simulink model "MyMotorCU_RTW"  (Simulink 7.5)
settings: Solver=ode1  SolverMode=SingleTasking  StartTime=0.0  StopTime=inf  FixedStep=0.0002  RelTol=1e-3
PreLoadFcn:
  | vehicle = 'Car'; if ~length(which('cmcmd')), cmenv; end
  | MyMotorCU_RTW_bus
InitFcn:
  | vehicle = 'Car'; if ~length(which('cmcmd')), cmenv; end
  | MyMotorCU_RTW_bus
libraries: simulink x6
Description:
  | CarMaker Real-Time Target (generic)
settings Model: Creator=ml  LastModifiedBy=ml
settings DebuggingCC: SolverPrmCheckMsg=none
settings HardwareCC: TargetHWDeviceType=32-bit Generic  ProdEqTarget=off
settings RTWCC: SystemTargetFile=CarMaker.tlc  TemplateMakefile=CarMaker_unix.tmf  Description=CarMaker Real-Time Target (32-bit)  ProcessScript=CarMaker_make_rtw_hook
settings CodeAppCC: MaxIdLength=63
settings STFCustomTargetCC: ModelReferenceCompliant=off  GeneratePreprocessorConditionals=Disable all  SystemTargetFile=CarMaker.tlc
settings GRTTargetCC: ModelReferenceCompliant=off  ParMdlRefBuildCompliant=off  CompOptLevelCompliant=off  MatFileLogging=off  ExtModeMexFile=noextcomm
settings CustomProperty: DataType=string  Value=..
settings EnumStrPairs: String=Car

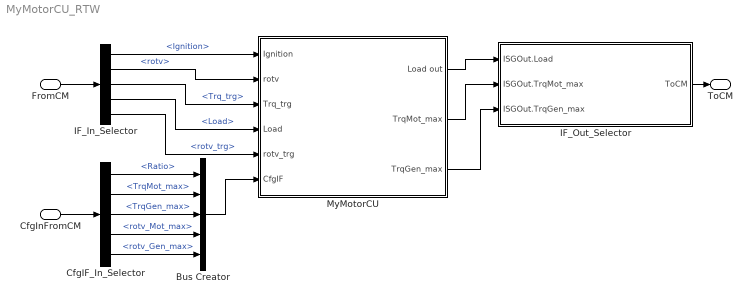
== system MyMotorCU_RTW ==
  FromCM : Inport  UseBusObject=on
      settings: BusObject=cmPTMotorCUIn
  CfgInFromCM : Inport  Port=2  UseBusObject=on
      settings: BusObject=cmPTMotorCUCfgIn
  Bus Creator : BusCreator  Inputs=5
  CfgIF_In_Selector : BusSelector  OutputSignals=ISG.Ratio,ISG.TrqMot_max,ISG.TrqGen_max,ISG.rotv_Mot_max,ISG.rotv_Gen_max
  IF_In_Selector : BusSelector  OutputSignals=Ignition,ISGIn.rotv,ISGIn.Trq_trg,ISGOut.Load,ISGIn.rotv_trg
  IF_Out_Selector : Subsystem
      settings: OpenFcn=cmSignalSelect('SignalSelection_CB',gcb)
      mask Type: Signal Selection
      mask Description: Signal Selection Block
  MyMotorCU : Subsystem
  ToCM : Outport  UseBusObject=on
      settings: BusObject=cmPTMotorCUOut
  wires:
  FromCM/1 -> IF_In_Selector/1
  IF_Out_Selector/1(ToCM) -> ToCM/1
  CfgInFromCM/1 -> CfgIF_In_Selector/1
  MyMotorCU/1(Load out) -> IF_Out_Selector/1(ISGOut.Load)
  MyMotorCU/2(TrqMot_max) -> IF_Out_Selector/2(ISGOut.TrqMot_max)
  MyMotorCU/3(TrqGen_max) -> IF_Out_Selector/3(ISGOut.TrqGen_max)
  IF_In_Selector/1 -> MyMotorCU/1(Ignition)  "<Ignition>"
  IF_In_Selector/2 -> MyMotorCU/2(rotv)  "<rotv>"
  IF_In_Selector/3 -> MyMotorCU/3(Trq_trg)  "<Trq_trg>"
  IF_In_Selector/4 -> MyMotorCU/4(Load)  "<Load>"
  IF_In_Selector/5 -> MyMotorCU/5(rotv_trg)  "<rotv_trg>"
  Bus Creator/1 -> MyMotorCU/6(CfgIF)
  CfgIF_In_Selector/1 -> Bus Creator/1  "<Ratio>"
  CfgIF_In_Selector/2 -> Bus Creator/2  "<TrqMot_max>"
  CfgIF_In_Selector/3 -> Bus Creator/3  "<TrqGen_max>"
  CfgIF_In_Selector/4 -> Bus Creator/4  "<rotv_Mot_max>"
  CfgIF_In_Selector/5 -> Bus Creator/5  "<rotv_Gen_max>"

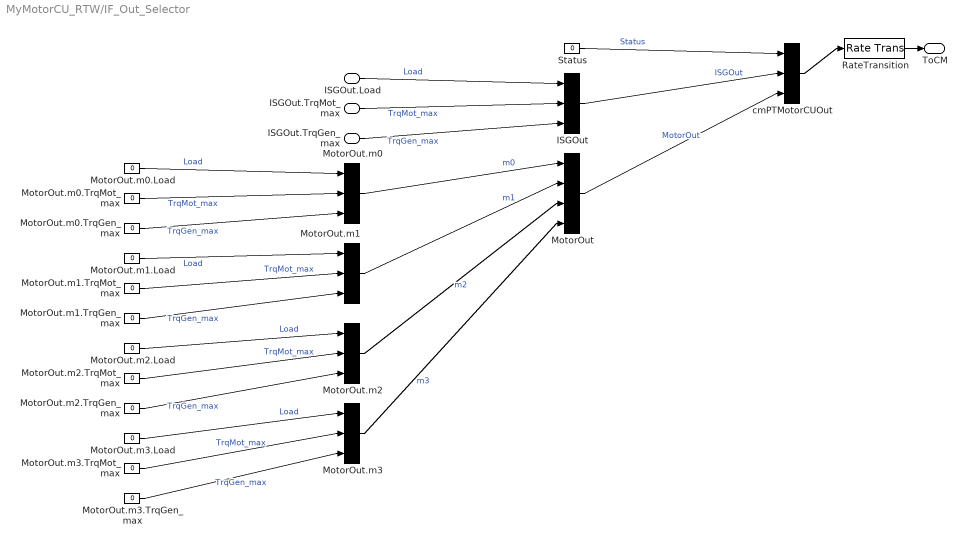
== system MyMotorCU_RTW/IF_Out_Selector ==
  ISGOut.Load : Inport
  ISGOut.TrqMot_max : Inport  Port=2
  ISGOut.TrqGen_max : Inport  Port=3
  ISGOut : BusCreator  Inputs=3
  MotorOut : BusCreator
  MotorOut.m{0..3} (4 alike) : BusCreator  Inputs=3
  MotorOut.m0.Load : Constant  Value=0
  MotorOut.m0.TrqGen_max : Constant  Value=0
  MotorOut.m0.TrqMot_max : Constant  Value=0
  MotorOut.m1.Load : Constant  Value=0
  MotorOut.m1.TrqGen_max : Constant  Value=0
  MotorOut.m1.TrqMot_max : Constant  Value=0
  MotorOut.m2.Load : Constant  Value=0
  MotorOut.m2.TrqGen_max : Constant  Value=0
  MotorOut.m2.TrqMot_max : Constant  Value=0
  MotorOut.m3.Load : Constant  Value=0
  MotorOut.m3.TrqGen_max : Constant  Value=0
  MotorOut.m3.TrqMot_max : Constant  Value=0
  RateTransition : RateTransition  OutPortSampleTime=str2num(get_param(bdroot,'FixedStep'))
  Status : Constant  Value=0
  cmPTMotorCUOut : BusCreator  Inputs=3
  ToCM : Outport
  wires:
  RateTransition/1 -> ToCM/1
  cmPTMotorCUOut/1 -> RateTransition/1
  Status/1 -> cmPTMotorCUOut/1  "Status"
  ISGOut/1 -> cmPTMotorCUOut/2  "ISGOut"
  MotorOut/1 -> cmPTMotorCUOut/3  "MotorOut"
  MotorOut.m0/1 -> MotorOut/1  "m0"
  MotorOut.m0.Load/1 -> MotorOut.m0/1  "Load"
  MotorOut.m0.TrqMot_max/1 -> MotorOut.m0/2  "TrqMot_max"
  MotorOut.m0.TrqGen_max/1 -> MotorOut.m0/3  "TrqGen_max"
  MotorOut.m1/1 -> MotorOut/2  "m1"
  MotorOut.m1.Load/1 -> MotorOut.m1/1  "Load"
  MotorOut.m1.TrqMot_max/1 -> MotorOut.m1/2  "TrqMot_max"
  MotorOut.m1.TrqGen_max/1 -> MotorOut.m1/3  "TrqGen_max"
  MotorOut.m2/1 -> MotorOut/3  "m2"
  MotorOut.m2.Load/1 -> MotorOut.m2/1  "Load"
  MotorOut.m2.TrqMot_max/1 -> MotorOut.m2/2  "TrqMot_max"
  MotorOut.m2.TrqGen_max/1 -> MotorOut.m2/3  "TrqGen_max"
  MotorOut.m3/1 -> MotorOut/4  "m3"
  MotorOut.m3.Load/1 -> MotorOut.m3/1  "Load"
  MotorOut.m3.TrqMot_max/1 -> MotorOut.m3/2  "TrqMot_max"
  MotorOut.m3.TrqGen_max/1 -> MotorOut.m3/3  "TrqGen_max"
  ISGOut.Load/1 -> ISGOut/1  "Load"
  ISGOut.TrqMot_max/1 -> ISGOut/2  "TrqMot_max"
  ISGOut.TrqGen_max/1 -> ISGOut/3  "TrqGen_max"

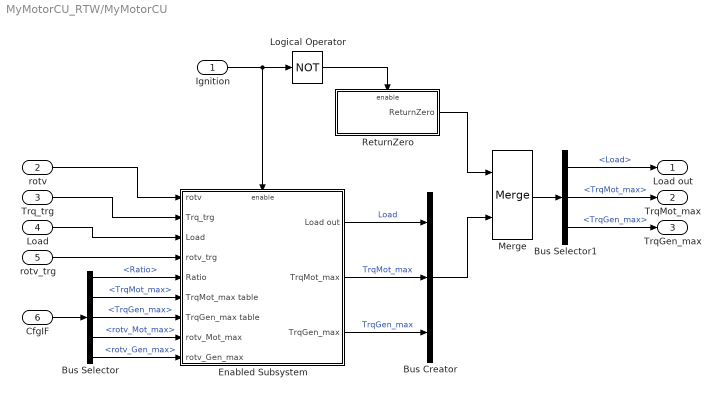
== system MyMotorCU_RTW/MyMotorCU ==
  Ignition : Inport  OutDataType=sfix(16)  OutScaling=2^0
  rotv : Inport  Port=2  OutDataType=sfix(16)  OutScaling=2^0
  Trq_trg : Inport  Port=3  OutDataType=sfix(16)  OutScaling=2^0
  Load : Inport  Port=4  OutDataType=sfix(16)  OutScaling=2^0
  rotv_trg : Inport  Port=5  OutDataType=sfix(16)  OutScaling=2^0
  CfgIF : Inport  Port=6  OutDataType=sfix(16)  OutScaling=2^0
  Bus Creator : BusCreator  Inputs=3
  Bus Selector : BusSelector  OutputSignals=Ratio,TrqMot_max,TrqGen_max,rotv_Mot_max,rotv_Gen_max
  Bus Selector1 : BusSelector  OutputSignals=Load,TrqMot_max,TrqGen_max
  Enabled Subsystem : Subsystem  TreatAsAtomicUnit=on
  Logical Operator : Logic  Operator=NOT  AllPortsSameDT=off  OutDataTypeMode=boolean  OutDataTypeStr=boolean
  Merge : Merge
  ReturnZero : Subsystem  TreatAsAtomicUnit=on
  Load out : Outport  OutDataType=sfix(16)  OutScaling=2^0
  TrqMot_max : Outport  Port=2  OutDataType=sfix(16)  OutScaling=2^0
  TrqGen_max : Outport  Port=3  OutDataType=sfix(16)  OutScaling=2^0
  wires:
  Ignition/1 -> Enabled Subsystem/Enable, Logical Operator/1
  Logical Operator/1 -> ReturnZero/Enable
  rotv/1 -> Enabled Subsystem/1(rotv)
  CfgIF/1 -> Bus Selector/1
  Bus Selector/1 -> Enabled Subsystem/5(Ratio)  "<Ratio>"
  Bus Selector/2 -> Enabled Subsystem/6(TrqMot_max table)  "<TrqMot_max>"
  Bus Selector/3 -> Enabled Subsystem/7(TrqGen_max table)  "<TrqGen_max>"
  Bus Selector/4 -> Enabled Subsystem/8(rotv_Mot_max)  "<rotv_Mot_max>"
  Bus Selector/5 -> Enabled Subsystem/9(rotv_Gen_max)  "<rotv_Gen_max>"
  Trq_trg/1 -> Enabled Subsystem/2(Trq_trg)
  Load/1 -> Enabled Subsystem/3(Load)
  rotv_trg/1 -> Enabled Subsystem/4(rotv_trg)
  Enabled Subsystem/1(Load out) -> Bus Creator/1  "Load"
  Enabled Subsystem/2(TrqMot_max) -> Bus Creator/2  "TrqMot_max"
  Enabled Subsystem/3(TrqGen_max) -> Bus Creator/3  "TrqGen_max"
  ReturnZero/1(ReturnZero) -> Merge/1
  Bus Creator/1 -> Merge/2
  Merge/1 -> Bus Selector1/1
  Bus Selector1/3 -> TrqGen_max/1  "<TrqGen_max>"
  Bus Selector1/2 -> TrqMot_max/1  "<TrqMot_max>"
  Bus Selector1/1 -> Load out/1  "<Load>"

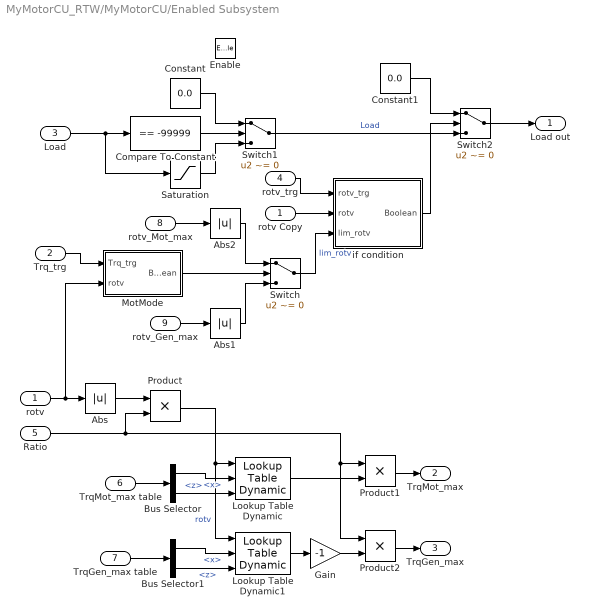
== system MyMotorCU_RTW/MyMotorCU/Enabled Subsystem ==
  rotv : Inport  OutDataType=sfix(16)  OutScaling=2^0
  Trq_trg : Inport  Port=2  OutDataType=sfix(16)  OutScaling=2^0
  Load : Inport  Port=3  OutDataType=sfix(16)  OutScaling=2^0
  rotv_trg : Inport  Port=4  OutDataType=sfix(16)  OutScaling=2^0
  Ratio : Inport  Port=5  OutDataType=sfix(16)  OutScaling=2^0
  TrqMot_max table : Inport  Port=6  OutDataType=sfix(16)  OutScaling=2^0
  TrqGen_max table : Inport  Port=7  OutDataType=sfix(16)  OutScaling=2^0
  rotv_Mot_max : Inport  Port=8  OutDataType=sfix(16)  OutScaling=2^0
  rotv_Gen_max : Inport  Port=9  OutDataType=sfix(16)  OutScaling=2^0
  Enable : EnablePort
  Abs : Abs  OutDataType=sfix(16)  OutScaling=2^0
  Abs1 : Abs  OutDataType=sfix(16)  OutScaling=2^0
  Abs2 : Abs  OutDataType=sfix(16)  OutScaling=2^0
  Bus Selector : BusSelector  OutputSignals=x,z
  Bus Selector1 : BusSelector  OutputSignals=x,z
  Compare To Constant : simulink/Logic and Bit Operations/Compare To Constant  SystemSampleTime=-1  relop===  const=-99999  LogicOutDataTypeMode=uint8  ZeroCross=off
  Constant : Constant  Value=0.0  OutDataType=sfix(16)  OutScaling=2^0
  Constant1 : Constant  Value=0.0  OutDataType=sfix(16)  OutScaling=2^0
  Gain : Gain  Gain=-1  ParameterDataType=sfix(16)  ParameterScaling=2^0  OutDataType=sfix(16)  OutScaling=2^0
  Lookup Table Dynamic : simulink/Lookup Tables/Lookup Table Dynamic  LookUpMeth=Interpolation-Use End Values  OutDataTypeStr=float('double')  OutputDataTypeScalingMode=Specify via dialog  OutDataType=float('double')  OutScaling=2^-10  DoSatur=off
  Lookup Table Dynamic1 : simulink/Lookup Tables/Lookup Table Dynamic  LookUpMeth=Interpolation-Use End Values  OutDataTypeStr=float('double')  OutputDataTypeScalingMode=Specify via dialog  OutDataType=float('double')  OutScaling=2^-10  DoSatur=off
  MotMode : Subsystem
  Product : Product  OutDataType=sfix(16)  OutScaling=2^0  RndMeth=Zero
  Product1 : Product  OutDataType=sfix(16)  OutScaling=2^0  RndMeth=Zero
  Product2 : Product  OutDataType=sfix(16)  OutScaling=2^0  RndMeth=Zero
  Saturation : Saturate  UpperLimit=1  LowerLimit=-1  OutDataType=sfix(16)  OutScaling=2^0
  Switch : Switch  Criteria=u2 ~= 0  OutDataType=sfix(16)  OutScaling=2^0
  Switch1 : Switch  Criteria=u2 ~= 0  OutDataType=sfix(16)  OutScaling=2^0
  Switch2 : Switch  Criteria=u2 ~= 0  OutDataType=sfix(16)  OutScaling=2^0
  if condition : Subsystem
  rotv Copy : InportShadow  Port=1  OutDataType=sfix(16)  OutScaling=2^0
  Load out : Outport  OutDataType=sfix(16)  OutScaling=2^0
  TrqMot_max : Outport  Port=2  OutDataType=sfix(16)  OutScaling=2^0
  TrqGen_max : Outport  Port=3  OutDataType=sfix(16)  OutScaling=2^0
  wires:
  rotv/1 -> Abs/1, MotMode/2(rotv)
  Ratio/1 -> Product/2, Product2/1, Product1/1
  Abs/1 -> Product/1
  TrqMot_max table/1 -> Bus Selector/1
  Bus Selector/1 -> Lookup Table Dynamic/2  "<x>"
  TrqGen_max table/1 -> Bus Selector1/1
  Bus Selector1/1 -> Lookup Table Dynamic1/2  "<x>"
  Bus Selector1/2 -> Lookup Table Dynamic1/3  "<z>"
  Lookup Table Dynamic1/1 -> Gain/1
  rotv_Gen_max/1 -> Abs1/1
  rotv_Mot_max/1 -> Abs2/1
  Switch/1 -> if condition/3(lim_rotv)  "lim_rotv"
  Product1/1 -> TrqMot_max/1
  Product2/1 -> TrqGen_max/1
  Gain/1 -> Product2/2
  MotMode/1(Boolean) -> Switch/2
  Trq_trg/1 -> MotMode/1(Trq_trg)
  Load/1 -> Compare To Constant/1, Saturation/1
  Compare To Constant/1 -> Switch1/2
  Constant/1 -> Switch1/1
  Saturation/1 -> Switch1/3
  Switch2/1 -> Load out/1
  Constant1/1 -> Switch2/1
  Switch1/1 -> Switch2/3  "Load"
  if condition/1(Boolean) -> Switch2/2
  rotv_trg/1 -> if condition/1(rotv_trg)
  Product/1 -> Lookup Table Dynamic/1, Lookup Table Dynamic1/1  "rotv"
  Abs1/1 -> Switch/3
  Abs2/1 -> Switch/1
  Lookup Table Dynamic/1 -> Product1/2
  Bus Selector/2 -> Lookup Table Dynamic/3  "<z>"
  rotv Copy/1 -> if condition/2(rotv)

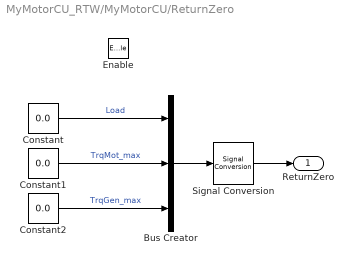
== system MyMotorCU_RTW/MyMotorCU/ReturnZero ==
  Enable : EnablePort
  Bus Creator : BusCreator  Inputs=3
  Constant : Constant  Value=0.0  OutDataType=sfix(16)  OutScaling=2^0
  Constant1 : Constant  Value=0.0  OutDataType=sfix(16)  OutScaling=2^0
  Constant2 : Constant  Value=0.0  OutDataType=sfix(16)  OutScaling=2^0
  Signal Conversion : SignalConversion  ConversionOutput=Bus copy
  ReturnZero : Outport  OutDataType=sfix(16)  OutScaling=2^0
  wires:
  Bus Creator/1 -> Signal Conversion/1
  Constant/1 -> Bus Creator/1  "Load"
  Constant1/1 -> Bus Creator/2  "TrqMot_max"
  Constant2/1 -> Bus Creator/3  "TrqGen_max"
  Signal Conversion/1 -> ReturnZero/1

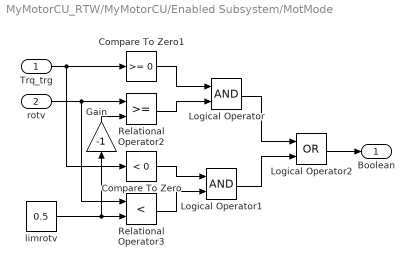
== system MyMotorCU_RTW/MyMotorCU/Enabled Subsystem/MotMode ==
  Trq_trg : Inport  OutDataType=sfix(16)  OutScaling=2^0
  rotv : Inport  Port=2  OutDataType=sfix(16)  OutScaling=2^0
  Compare To Zero : simulink/Logic and Bit Operations/Compare To Zero  SystemSampleTime=-1  relop=<  LogicOutDataTypeMode=uint8  ZeroCross=off
  Compare To Zero1 : simulink/Logic and Bit Operations/Compare To Zero  SystemSampleTime=-1  relop=>=  LogicOutDataTypeMode=uint8  ZeroCross=off
  Gain : Gain  Gain=-1  ParameterDataType=sfix(16)  ParameterScaling=2^0  OutDataType=sfix(16)  OutScaling=2^0
  Logical Operator : Logic  AllPortsSameDT=off  OutDataTypeMode=boolean  OutDataTypeStr=boolean
  Logical Operator1 : Logic  AllPortsSameDT=off  OutDataTypeMode=boolean  OutDataTypeStr=boolean
  Logical Operator2 : Logic  Operator=OR  AllPortsSameDT=off  OutDataTypeMode=boolean  OutDataTypeStr=boolean
  Relational Operator2 : RelationalOperator  LogicOutDataTypeMode=boolean  OutDataTypeStr=boolean
  Relational Operator3 : RelationalOperator  Operator=<  LogicOutDataTypeMode=boolean  OutDataTypeStr=boolean
  limrotv : Constant  Value=0.5  OutDataType=sfix(16)  OutScaling=2^0
  Boolean : Outport  OutDataType=sfix(16)  OutScaling=2^0
  wires:
  Logical Operator2/1 -> Boolean/1
  Logical Operator/1 -> Logical Operator2/1
  Logical Operator1/1 -> Logical Operator2/2
  Compare To Zero1/1 -> Logical Operator/1
  Trq_trg/1 -> Compare To Zero1/1, Compare To Zero/1
  Compare To Zero/1 -> Logical Operator1/1
  Relational Operator2/1 -> Logical Operator/2
  rotv/1 -> Relational Operator2/1, Relational Operator3/1
  limrotv/1 -> Relational Operator3/2, Gain/1
  Relational Operator3/1 -> Logical Operator1/2
  Gain/1 -> Relational Operator2/2

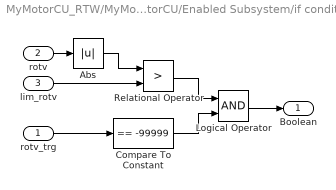
== system MyMotorCU_RTW/MyMotorCU/Enabled Subsystem/if condition ==
  rotv_trg : Inport  OutDataType=sfix(16)  OutScaling=2^0
  rotv : Inport  Port=2  OutDataType=sfix(16)  OutScaling=2^0
  lim_rotv : Inport  Port=3  OutDataType=sfix(16)  OutScaling=2^0
  Abs : Abs  OutDataType=sfix(16)  OutScaling=2^0
  Compare To Constant : simulink/Logic and Bit Operations/Compare To Constant  SystemSampleTime=-1  relop===  const=-99999  LogicOutDataTypeMode=boolean  ZeroCross=off
  Logical Operator : Logic  AllPortsSameDT=off  OutDataTypeMode=boolean  OutDataTypeStr=boolean
  Relational Operator : RelationalOperator  Operator=>  LogicOutDataTypeMode=boolean  OutDataTypeStr=boolean
  Boolean : Outport  OutDataType=sfix(16)  OutScaling=2^0
  wires:
  Logical Operator/1 -> Boolean/1
  rotv_trg/1 -> Compare To Constant/1
  Compare To Constant/1 -> Logical Operator/2
  Relational Operator/1 -> Logical Operator/1
  lim_rotv/1 -> Relational Operator/2
  rotv/1 -> Abs/1
  Abs/1 -> Relational Operator/1
